simulink model "Inverted_Pend_Lab"  (R2021a)
settings: Solver=VariableStepAuto  StartTime=0.0  StopTime=50  MaxStep=1e-3  RelTol=1e-9
values from neighbouring files (symbols this model uses):
  B = 7.1600e-05    (= 7.16e-05)    [Lab_Startup_Script.m]
  Bs = (2000*pi*0.9)/(10)    (= 565.486677646)    [Lab_Startup_Script.m]
  Bw = 7.1700e-05    (= 7.17e-05)    [Lab_Startup_Script.m]
  distance = 4    [Lab_Startup_Script.m]
  g = 9.8    [Lab_Startup_Script.m]
  JBs = MBs*0.5*(Bsd/2)^2    (= 4.09817752346e-05)    [Lab_Startup_Script.m]
  Jm = 4 * 10 ^ (-6)    (= 4e-06)    [Lab_Startup_Script.m]
  Jr = (1/3)*m*(l*2)^2    (= 0.000666666666667)    [Lab_Startup_Script.m]
  Jw = 0.5*Mw*wR^2    (= 4.59960580412e-05)    [Lab_Startup_Script.m]
  Kb = 13.2/(3000*2*pi/60)    (= 0.0420169049763)    [Lab_Startup_Script.m]
  Km = 42*10^(-3)    (= 0.042)    [Lab_Startup_Script.m]
  l = 0.1    [Lab_Startup_Script.m]
  La = 1.16*10^(-3)    (= 0.00116)    [Lab_Startup_Script.m]
  m = 0.05    [Lab_Startup_Script.m]
  Mt = M  + m    (= 1.05)    [Lab_Startup_Script.m]
  openSec = 0.07    [Lab_Startup_Script.m]
  pinDistance = 2    [Lab_Startup_Script.m]
  Ra = 8.4    [Lab_Startup_Script.m]
  RPM = 3*60    (= 180)    [Lab_Startup_Script.m]
  startDelay = (1/(RPM/60))*(1/numSection)*(1+openSec*0.5) - mod(timeToWheel,(1/(RPM/60))*(1/numSection))    [Lab_Startup_Script.m]
libraries: pid_lib x3, dspswit3 x2
settings Model: Creator=Chris  LastModifiedBy=Chris

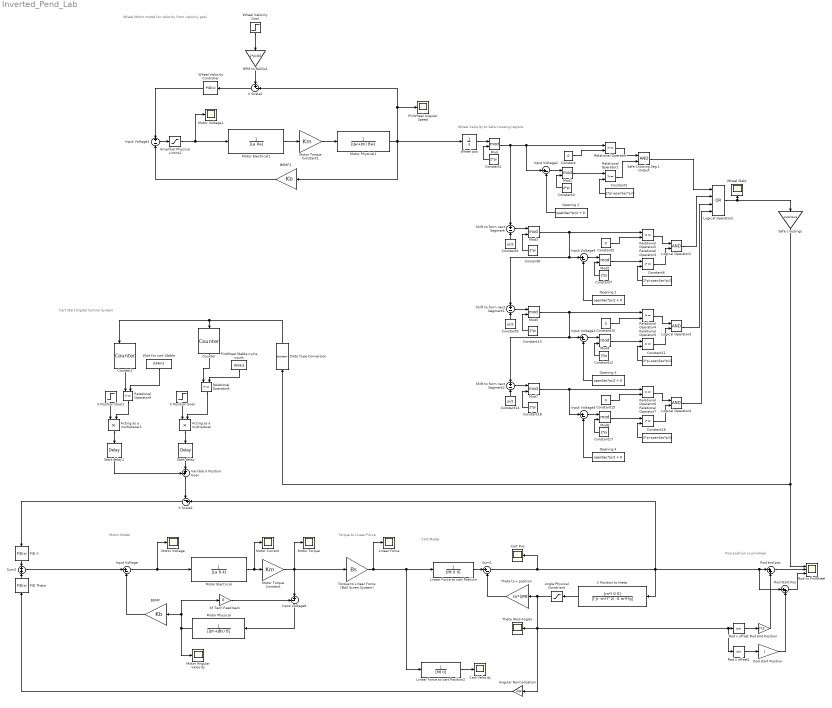
== system Inverted_Pend_Lab ==
  note: Cart Start Digital Control System
  note: Wheel Velocity to Safe crossing regions
  note: Wheel Motor model for velocity from velocity goal
  note: Rod position vs pinwheel
  note: Cart Model
  note: Torque to Linear Force
  note: Motor Model
  Acting as a multiplexer : Product
  Acting as a multiplexer1 : Product
  Amplifier Physical Limits1 : Saturate  UpperLimit=18  LowerLimit=-18
  Angle Physical Constriant : Saturate  UpperLimit=pi/2  LowerLimit=-pi/2
  Angular Normalization : Gain  Gain=2/pi
  BEMF : Gain  Gain=Kb
  BEMF1 : Gain  Gain=Kb
  Cart Pos : Scope
  Cart Velocity : Scope
  Consant8 : Constant  Value=2*pi
  Constant{,5,10,15} (4 alike) : Constant  Value=0
  Constant{1,3,7,12..13,17..18} (7 alike) : Constant  Value=2*pi
  Constant{2,6,11,16} (4 alike) : Constant  Value=2*pi-openSec*pi/2
  Constant14 : Constant  Value=pi/2
  Constant4 : Constant  Value=pi/2
  Constant9 : Constant  Value=pi/2
  Counter : dspswit3/Counter  Direction=Up  CountEvent=Rising edge  CounterSize=32 bits  MaxCount=255  InitialCount=0  Output=Count  HitValue=32  ResetInput=off  SamplesPerFrame=1  Ts=1  CntDtype=uint32  HitDtype=Logical
  Counter1 : dspswit3/Counter  Direction=Up  CountEvent=Rising edge  CounterSize=32 bits  MaxCount=255  InitialCount=0  Output=Count  HitValue=32  ResetInput=on  SamplesPerFrame=1  Ts=1  CntDtype=uint32  HitDtype=Logical
  Data Type Conversion : DataTypeConversion  OutDataTypeStr=boolean
  Input Voltage{,2..5} (5 alike) : Sum  Inputs=|+-
  Input Voltage1 : Sum  Inputs=+-
  Input Voltage6 : Sum  Inputs=-+|
  Kf Tach Feed back : Gain  Gain=0
  Linear Force : Scope
  Linear Force to cart Position : TransferFcn  Denominator=[Mt 0 0]
  Linear Force to cart Position2 : TransferFcn  Denominator=[Mt 0]
  Logical Operator1 : Logic  AllPortsSameDT=off  OutDataTypeStr=boolean
  Logical Operator2 : Logic  Operator=OR  Inputs=4  AllPortsSameDT=off  OutDataTypeStr=boolean
  Logical Operator3 : Logic  AllPortsSameDT=off  OutDataTypeStr=boolean
  Logical Operator4 : Logic  AllPortsSameDT=off  OutDataTypeStr=boolean
  Mod{,1..7} (8 alike) : Math  Operator=mod  SaturateOnIntegerOverflow=on
  Motor Angular Velocity : Scope
  Motor Current : Scope
  Motor Electrical : TransferFcn  Denominator=[La 8.4]
  Motor Electrical1 : TransferFcn  Denominator=[La Ra]
  Motor Physical : TransferFcn  Denominator=[(Jm+JBs) B]
  Motor Physical1 : TransferFcn  Denominator=[(Jw+Jm) Bw]
  Motor Torque : Scope
  Motor Torque Constant : Gain  Gain=Km
  Motor Torque Constant1 : Gain  Gain=Km
  Motor Voltage : Scope
  Motor Voltage1 : Scope
  Opening {1..4} (4 alike) : Constant  Value=openSec*pi/2 + 0
  PID Theta : pid_lib/PID Controller  Controller=PID  Form=Parallel  TimeDomain=Continuous-time  UseExternalTs=off  SampleTime=-1  IntegratorMethod=Forward Euler  FilterMethod=Forward Euler  ControllerParametersSource=internal  P=400  I=150  D=10  UseFilter=on  N=200  TunerSelectOption=Transfer Function Based (PID Tuner App)  InitialConditionSource=internal  InitialConditionForIntegrator=0  InitialConditionForFilter=0  DifferentiatorICPrevScaledInput=0  ExternalReset=none  TrackingMode=off  Kt=1  LimitOutput=off  SatLimitsSource=internal  UpperSaturationLimit=inf  LowerSaturationLimit=-inf  LinearizeAsGain=on  AntiWindupMode=none  Kb=1  POutMin=[]  POutMax=[]  IOutMin=[]  IOutMax=[]  DOutMin=[]  DOutMax=[]  NOutMin=[]  NOutMax=[]  SumOutMin=[]  SumOutMax=[]  SaturationOutMin=[]  SaturationOutMax=[]  PParamMin=[]  PParamMax=[]  IParamMin=[]  IParamMax=[]  DParamMin=[]  DParamMax=[]  NParamMin=[]  NParamMax=[]  KbParamMin=[]  KbParamMax=[]  KtParamMin=[]  KtParamMax=[]  KbOutMin=[]  KbOutMax=[]  KtOutMin=[]  KtOutMax=[]  IntegratorOutMin=[]  IntegratorOutMax=[]  FilterOutMin=[]  FilterOutMax=[]  SumI1OutMin=[]  SumI1OutMax=[]  SumI2OutMin=[]  SumI2OutMax=[]  SumI3OutMin=[]  SumI3OutMax=[]  SumI4OutMin=[]  SumI4OutMax=[]  SumDOutMin=[]  SumDOutMax=[]  DifferentiatorOutMin=[]  DifferentiatorOutMax=[]  FilterDiffOutCoefMin=[]  FilterDiffOutCoefMax=[]  ReciprocalOutMin=[]  ReciprocalOutMax=[]  SumDenOutMin=[]  SumDenOutMax=[]  SumNumOutMin=[]  SumNumOutMax=[]  DivideOutMin=[]  DivideOutMax=[]  UdiffTsProdOutMin=[]  UdiffTsProdOutMax=[]  NTsProdOutMin=[]  NTsProdOutMax=[]  UintegralTsProdOutMin=[]  UintegralTsProdOutMax=[]  UngainTsProdOutMin=[]  UngainTsProdOutMax=[]  IntegratorContinuousStateAttributes=''  IntegratorStateMustResolveToSignalObject=off  IntegratorRTWStateStorageClass=Auto  FilterContinuousStateAttributes=''  FilterStateMustResolveToSignalObject=off  FilterRTWStateStorageClass=Auto  ParallelPVariant=InternalParameters  IdealPVariant=Disabled  IVariant=InternalParameters  DVariant=InternalParameters  IntegratorVariant=Continuous  SatVariant=Disabled  AWVariant=Passthrough  PCopyVariant=Disabled  TRVariant=Disabled  FdbkBlocksVariant=Forward  IdealPFdbkVariant=Disabled  SatFdbkVariant=Disabled  DerivativeFilterVariant=ContFilter  NVariant=InternalParameters  NCopyVariant=Disabled  FilterICVariant=InternalICsFilter  IntegratorICVariant=InternalICs  ExternalResetVariant=Disabled  TRSumVariant=Passthrough  SumFdbkVariant=Disabled  SumVariant=Sum_PID  TsampFilterVariant=InternalTs  TsampNgainVariant=Passthrough  TsampIntegralVariant=Passthrough  ExternalSaturationOutDataTypeStr=Inherit: Same as second input
  PID X : pid_lib/PID Controller  Controller=PID  Form=Parallel  TimeDomain=Continuous-time  UseExternalTs=off  SampleTime=-1  IntegratorMethod=Forward Euler  FilterMethod=Forward Euler  ControllerParametersSource=internal  P=2.4  I=0  D=2  UseFilter=on  N=1  TunerSelectOption=Transfer Function Based (PID Tuner App)  InitialConditionSource=internal  InitialConditionForIntegrator=0  InitialConditionForFilter=0  DifferentiatorICPrevScaledInput=0  ExternalReset=none  TrackingMode=off  Kt=1  LimitOutput=off  SatLimitsSource=internal  UpperSaturationLimit=inf  LowerSaturationLimit=-inf  LinearizeAsGain=on  AntiWindupMode=none  Kb=1  POutMin=[]  POutMax=[]  IOutMin=[]  IOutMax=[]  DOutMin=[]  DOutMax=[]  NOutMin=[]  NOutMax=[]  SumOutMin=[]  SumOutMax=[]  SaturationOutMin=[]  SaturationOutMax=[]  PParamMin=[]  PParamMax=[]  IParamMin=[]  IParamMax=[]  DParamMin=[]  DParamMax=[]  NParamMin=[]  NParamMax=[]  KbParamMin=[]  KbParamMax=[]  KtParamMin=[]  KtParamMax=[]  KbOutMin=[]  KbOutMax=[]  KtOutMin=[]  KtOutMax=[]  IntegratorOutMin=[]  IntegratorOutMax=[]  FilterOutMin=[]  FilterOutMax=[]  SumI1OutMin=[]  SumI1OutMax=[]  SumI2OutMin=[]  SumI2OutMax=[]  SumI3OutMin=[]  SumI3OutMax=[]  SumI4OutMin=[]  SumI4OutMax=[]  SumDOutMin=[]  SumDOutMax=[]  DifferentiatorOutMin=[]  DifferentiatorOutMax=[]  FilterDiffOutCoefMin=[]  FilterDiffOutCoefMax=[]  ReciprocalOutMin=[]  ReciprocalOutMax=[]  SumDenOutMin=[]  SumDenOutMax=[]  SumNumOutMin=[]  SumNumOutMax=[]  DivideOutMin=[]  DivideOutMax=[]  UdiffTsProdOutMin=[]  UdiffTsProdOutMax=[]  NTsProdOutMin=[]  NTsProdOutMax=[]  UintegralTsProdOutMin=[]  UintegralTsProdOutMax=[]  UngainTsProdOutMin=[]  UngainTsProdOutMax=[]  IntegratorContinuousStateAttributes=''  IntegratorStateMustResolveToSignalObject=off  IntegratorRTWStateStorageClass=Auto  FilterContinuousStateAttributes=''  FilterStateMustResolveToSignalObject=off  FilterRTWStateStorageClass=Auto  ParallelPVariant=InternalParameters  IdealPVariant=Disabled  IVariant=InternalParameters  DVariant=InternalParameters  IntegratorVariant=Continuous  SatVariant=Disabled  AWVariant=Passthrough  PCopyVariant=Disabled  TRVariant=Disabled  FdbkBlocksVariant=Forward  IdealPFdbkVariant=Disabled  SatFdbkVariant=Disabled  DerivativeFilterVariant=ContFilter  NVariant=InternalParameters  NCopyVariant=Disabled  FilterICVariant=InternalICsFilter  IntegratorICVariant=InternalICs  ExternalResetVariant=Disabled  TRSumVariant=Passthrough  SumFdbkVariant=Disabled  SumVariant=Sum_PID  TsampFilterVariant=InternalTs  TsampNgainVariant=Passthrough  TsampIntegralVariant=Passthrough  ExternalSaturationOutDataTypeStr=Inherit: Same as second input
  PinWheel Angular Speed : Scope
  PinWheel Stable cycle count : Constant  Value=RPM/3
  RPM to RAD/s1 : Gain  Gain=2*pi/60
  Relational Operator{,1..9} (10 alike) : RelationalOperator  OutDataTypeStr=boolean  RndMeth=Simplest
  Rod End Position : Gain  Gain=l*2
  Rod Start Pos : Sum  Inputs=|++
  Rod end pos : Sum  Inputs=|++
  Rod start Position : Gain  Gain=l
  Rod vs PinWheel : Scope  NumInputPorts=3
  Rod x offset : Trigonometry
  Rod x offset1 : Trigonometry
  Safe Crossing Seg 1 Output : Logic  AllPortsSameDT=off  OutDataTypeStr=boolean
  Safe crossings : Gain  Gain=pinDistance
  Shift to form next Segment : Sum  Inputs=+-
  Shift to form next Segment1 : Sum  Inputs=+-
  Shift to form next Segment2 : Sum  Inputs=+-
  Start delay : TransportDelay  DelayTime=startDelay
  Start delay1 : TransportDelay  DelayTime=startDelay
  Sum1 : Sum  Inputs=|+-
  Sum3 : Sum
  Theta (Rod Angle) : Scope
  "Theta to x position " : Gain  Gain=m*l/Mt
  Torque to Linear Force (Ball Screw System) : Gain  Gain=Bs
  Varrible X Position Goal : Sum  Inputs=++|
  Wait for cart Stable : Constant  Value=RPM*2
  Wheel Slats : Scope
  Wheel Velocity Controller : pid_lib/PID Controller  Controller=PID  Form=Parallel  TimeDomain=Continuous-time  UseExternalTs=off  SampleTime=-1  IntegratorMethod=Forward Euler  FilterMethod=Forward Euler  ControllerParametersSource=internal  P=1  I=1  D=0  UseFilter=on  N=0  TunerSelectOption=Transfer Function Based (PID Tuner App)  InitialConditionSource=internal  InitialConditionForIntegrator=0  InitialConditionForFilter=0  DifferentiatorICPrevScaledInput=0  ExternalReset=none  TrackingMode=off  Kt=1  LimitOutput=off  SatLimitsSource=internal  UpperSaturationLimit=inf  LowerSaturationLimit=-inf  LinearizeAsGain=on  AntiWindupMode=none  Kb=1  POutMin=[]  POutMax=[]  IOutMin=[]  IOutMax=[]  DOutMin=[]  DOutMax=[]  NOutMin=[]  NOutMax=[]  SumOutMin=[]  SumOutMax=[]  SaturationOutMin=[]  SaturationOutMax=[]  PParamMin=[]  PParamMax=[]  IParamMin=[]  IParamMax=[]  DParamMin=[]  DParamMax=[]  NParamMin=[]  NParamMax=[]  KbParamMin=[]  KbParamMax=[]  KtParamMin=[]  KtParamMax=[]  KbOutMin=[]  KbOutMax=[]  KtOutMin=[]  KtOutMax=[]  IntegratorOutMin=[]  IntegratorOutMax=[]  FilterOutMin=[]  FilterOutMax=[]  SumI1OutMin=[]  SumI1OutMax=[]  SumI2OutMin=[]  SumI2OutMax=[]  SumI3OutMin=[]  SumI3OutMax=[]  SumI4OutMin=[]  SumI4OutMax=[]  SumDOutMin=[]  SumDOutMax=[]  DifferentiatorOutMin=[]  DifferentiatorOutMax=[]  FilterDiffOutCoefMin=[]  FilterDiffOutCoefMax=[]  ReciprocalOutMin=[]  ReciprocalOutMax=[]  SumDenOutMin=[]  SumDenOutMax=[]  SumNumOutMin=[]  SumNumOutMax=[]  DivideOutMin=[]  DivideOutMax=[]  UdiffTsProdOutMin=[]  UdiffTsProdOutMax=[]  NTsProdOutMin=[]  NTsProdOutMax=[]  UintegralTsProdOutMin=[]  UintegralTsProdOutMax=[]  UngainTsProdOutMin=[]  UngainTsProdOutMax=[]  IntegratorContinuousStateAttributes=''  IntegratorStateMustResolveToSignalObject=off  IntegratorRTWStateStorageClass=Auto  FilterContinuousStateAttributes=''  FilterStateMustResolveToSignalObject=off  FilterRTWStateStorageClass=Auto  ParallelPVariant=InternalParameters  IdealPVariant=Disabled  IVariant=InternalParameters  DVariant=InternalParameters  IntegratorVariant=Continuous  SatVariant=Disabled  AWVariant=Passthrough  PCopyVariant=Disabled  TRVariant=Disabled  FdbkBlocksVariant=Forward  IdealPFdbkVariant=Disabled  SatFdbkVariant=Disabled  DerivativeFilterVariant=ContFilter  NVariant=InternalParameters  NCopyVariant=Disabled  FilterICVariant=InternalICsFilter  IntegratorICVariant=InternalICs  ExternalResetVariant=Disabled  TRSumVariant=Passthrough  SumFdbkVariant=Disabled  SumVariant=Sum_PID  TsampFilterVariant=InternalTs  TsampNgainVariant=Passthrough  TsampIntegralVariant=Passthrough  ExternalSaturationOutDataTypeStr=Inherit: Same as second input
  Wheel Velocity Goal : Step  Time=0  After=RPM  SampleTime=0
  Wheel pos : TransferFcn  Denominator=[1 0]
  X Position Goal : Step  Time=0  After=distance  SampleTime=0
  X Position Goal1 : Step  Time=0  After=-distance  SampleTime=0
  X Position to theta : TransferFcn  Numerator=[m*l 0 0]  Denominator="[(-Jr -m*l^2)  0 m*l*g]"
  X Scale1 : Sum  Inputs=-+|
  X Scale2 : Sum  Inputs=+-|
  wires:
  Motor Electrical/1 -> Motor Current/1, Motor Torque Constant/1
  Motor Physical/1 -> Kf Tach Feed back/1, BEMF/1, Motor Angular Velocity/1
  Input Voltage/1 -> Motor Voltage/1, Motor Electrical/1
  Motor Torque Constant/1 -> Torque to Linear Force (Ball Screw System)/1, Input Voltage6/2, Motor Torque/1
  Torque to Linear Force (Ball Screw System)/1 -> Linear Force to cart Position2/1, Linear Force to cart Position/1, Linear Force/1
  "Theta to x position "/1 -> Sum1/2
  Linear Force to cart Position/1 -> Sum1/1
  BEMF/1 -> Input Voltage/2
  X Position to theta/1 -> Angle Physical Constriant/1
  Sum1/1 -> Cart Pos/1, Rod Start Pos/1, Rod end pos/1, X Position to theta/1, X Scale1/2
  Rod x offset/1 -> Rod End Position/1
  Rod End Position/1 -> Rod end pos/2
  Rod end pos/1 -> Rod vs PinWheel/2
  Motor Electrical1/1 -> Motor Torque Constant1/1
  Input Voltage1/1 -> Amplifier Physical Limits1/1
  Motor Torque Constant1/1 -> Motor Physical1/1
  BEMF1/1 -> Input Voltage1/2
  Motor Physical1/1 -> BEMF1/1, Wheel pos/1, PinWheel Angular Speed/1, X Scale2/2
  X Scale2/1 -> Wheel Velocity Controller/1
  Wheel Velocity Goal/1 -> RPM to RAD/s1/1
  RPM to RAD/s1/1 -> X Scale2/1
  Amplifier Physical Limits1/1 -> Motor Voltage1/1, Motor Electrical1/1
  Constant1/1 -> Mod/2
  Mod/1 -> Shift to form next Segment/1, Relational Operator/1, Input Voltage2/1
  Relational Operator/1 -> Safe Crossing Seg 1 Output/1
  Relational Operator1/1 -> Safe Crossing Seg 1 Output/2
  Wheel pos/1 -> Mod/1
  Constant/1 -> Relational Operator/2
  Constant2/1 -> Relational Operator1/2
  Opening 1/1 -> Input Voltage2/2
  Input Voltage2/1 -> Mod1/1
  Mod1/1 -> Relational Operator1/1
  Constant3/1 -> Mod1/2
  Constant4/1 -> Shift to form next Segment/2
  Input Voltage4/1 -> Mod2/1
  Opening 2/1 -> Input Voltage4/2
  Relational Operator3/1 -> Logical Operator1/2
  Relational Operator2/1 -> Logical Operator1/1
  Constant5/1 -> Relational Operator2/2
  Constant6/1 -> Relational Operator3/2
  Constant7/1 -> Mod2/2
  Mod2/1 -> Relational Operator3/1
  Mod3/1 -> Relational Operator2/1, Shift to form next Segment1/1, Input Voltage4/1
  Consant8/1 -> Mod3/2
  Shift to form next Segment/1 -> Mod3/1
  Safe Crossing Seg 1 Output/1 -> Logical Operator2/1
  Logical Operator1/1 -> Logical Operator2/2
  Mod5/1 -> Relational Operator4/1, Input Voltage3/1, Shift to form next Segment2/1
  Constant9/1 -> Shift to form next Segment1/2
  Shift to form next Segment1/1 -> Mod5/1
  Constant12/1 -> Mod4/2
  Input Voltage3/1 -> Mod4/1
  Constant13/1 -> Mod5/2
  Relational Operator4/1 -> Logical Operator3/1
  Constant10/1 -> Relational Operator4/2
  Relational Operator5/1 -> Logical Operator3/2
  Opening 3/1 -> Input Voltage3/2
  Constant11/1 -> Relational Operator5/2
  Mod4/1 -> Relational Operator5/1
  Logical Operator3/1 -> Logical Operator2/3
  Mod7/1 -> Relational Operator6/1, Input Voltage5/1
  Constant14/1 -> Shift to form next Segment2/2
  Shift to form next Segment2/1 -> Mod7/1
  Constant17/1 -> Mod6/2
  Input Voltage5/1 -> Mod6/1
  Constant18/1 -> Mod7/2
  Relational Operator6/1 -> Logical Operator4/1
  Constant15/1 -> Relational Operator6/2
  Relational Operator7/1 -> Logical Operator4/2
  Opening 4/1 -> Input Voltage5/2
  Constant16/1 -> Relational Operator7/2
  Mod6/1 -> Relational Operator7/1
  Logical Operator4/1 -> Logical Operator2/4
  Acting as a multiplexer/1 -> Start delay/1
  X Position Goal/1 -> Acting as a multiplexer/1
  Relational Operator8/1 -> Acting as a multiplexer/2
  Counter/1 -> Relational Operator8/1
  PinWheel Stable cycle count/1 -> Relational Operator8/2
  Logical Operator2/1 -> Safe crossings/1, Wheel Slats/1
  Safe crossings/1 -> Rod vs PinWheel/1, Data Type Conversion/1
  Linear Force to cart Position2/1 -> Cart Velocity/1
  Acting as a multiplexer1/1 -> Start delay1/1
  Counter1/1 -> Relational Operator9/1
  Wait for cart Stable/1 -> Relational Operator9/2
  X Position Goal1/1 -> Acting as a multiplexer1/1
  Relational Operator9/1 -> Acting as a multiplexer1/2
  Start delay/1 -> Varrible X Position Goal/2
  Data Type Conversion/1 -> Counter1/1, Counter/1
  Rod start Position/1 -> Rod Start Pos/2
  Rod x offset1/1 -> Rod start Position/1
  Rod Start Pos/1 -> Rod vs PinWheel/3
  PID Theta/1 -> Sum3/2
  PID X/1 -> Sum3/1
  Angular Normalization/1 -> PID Theta/1
  Angle Physical Constriant/1 -> Rod x offset1/1, Rod x offset/1, Angular Normalization/1, Theta (Rod Angle)/1, "Theta to x position "/1
  Start delay1/1 -> Varrible X Position Goal/1
  Kf Tach Feed back/1 -> Input Voltage6/1
  Input Voltage6/1 -> Motor Physical/1
  X Scale1/1 -> PID X/1
  Sum3/1 -> Input Voltage/1
  Varrible X Position Goal/1 -> X Scale1/1
  Wheel Velocity Controller/1 -> Input Voltage1/1
